simulink model "Option2_Variable"  (R2023b)
settings: Solver=VariableStepAuto  StartTime=0.0  StopTime=25  FixedStep=dT  RelTol=1e-3
values from neighbouring files (symbols this model uses):
  a = A(A_index)    [Part2.m]
  Bc = B1 + B2    (= 2)    [Part2.m]
  Jc = J1 + J2    (= 101)    [Part2.m]
settings Model: Creator=joshc  LastModifiedBy=huert

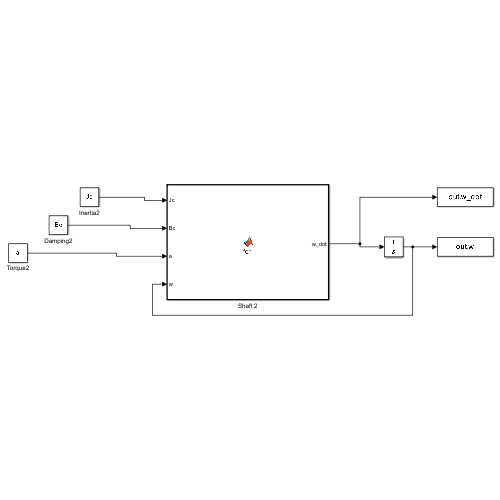
[thumbnail: Simulink's stored preview of the top-level diagram]
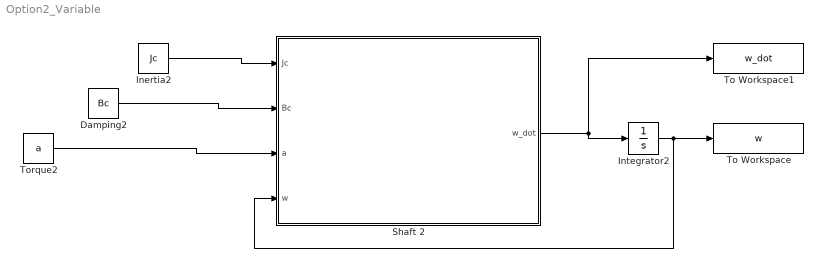
== system Option2_Variable ==
  Damping2 : Constant  Value=Bc
  Inertia2 : Constant  Value=Jc
  Integrator2 : Integrator  UpperSaturationLimit=1000
  Shaft 2 : MATLAB Function  TreatAsAtomicUnit=on
  To Workspace : ToWorkspace  VariableName=w  SaveFormat=Structure With Time  SampleTime=-1
  To Workspace1 : ToWorkspace  VariableName=w_dot  SaveFormat=Structure With Time  SampleTime=-1
  Torque2 : Constant  Value=a
  wires:
  Integrator2/1 -> Shaft 2/4(w), To Workspace/1
  Shaft 2/1(w_dot) -> To Workspace1/1, Integrator2/1
  Torque2/1 -> Shaft 2/3(a)
  Damping2/1 -> Shaft 2/2(Bc)
  Inertia2/1 -> Shaft 2/1(Jc)

== matlab function Option2_Variable/Shaft 2 ==
  data: Jc input; w_dot output; Bc input; a input; w input
function w_dot = fcn(Jc, Bc, a, w)

w_dot = (1/Jc)*(a - Bc*w);

end
